simulink model "BCM2_4"  (R2021b)
settings: Solver=FixedStepDiscrete  StartTime=0.0  StopTime=1  FixedStep=0.001  RelTol=1e-3  EnableMultiTasking=on
InitFcn:
  | mbd_mpc_consistency_checks(bdroot(gcs));
model workspace (MAT data in the model file):
  CAN_rec : Simulink.Signal (value not decoded)
  CAN_transm_stat : Simulink.Signal (value not decoded)
  CAN_trm : Simulink.Signal (value not decoded)
  DITHER_CFB0 : Simulink.Parameter (value not decoded)
  DITHER_CFB1 : Simulink.Parameter (value not decoded)
  DITHER_CFB2 : Simulink.Parameter (value not decoded)
  DITHER_EN0 : Simulink.Parameter (value not decoded)
  DITHER_EN1 : Simulink.Parameter (value not decoded)
  DITHER_EN2 : Simulink.Parameter (value not decoded)
  DITHER_SIZE0 : Simulink.Parameter (value not decoded)
  DITHER_SIZE1 : Simulink.Parameter (value not decoded)
  DITHER_SIZE2 : Simulink.Parameter (value not decoded)
  DITHER_STEP0 : Simulink.Parameter (value not decoded)
  DITHER_STEP1 : Simulink.Parameter (value not decoded)
  DITHER_STEP2 : Simulink.Parameter (value not decoded)
  DITHER_SYNC0 : Simulink.Parameter (value not decoded)
  DITHER_SYNC1 : Simulink.Parameter (value not decoded)
  DITHER_SYNC2 : Simulink.Parameter (value not decoded)
  ECUMbut : Simulink.Signal (value not decoded)
  FAULTN : Simulink.Signal (value not decoded)
  FM0 : Simulink.Parameter (value not decoded)
  FM1 : Simulink.Parameter (value not decoded)
  FM2 : Simulink.Parameter (value not decoded)
  FME : Simulink.Parameter (value not decoded)
  Fsys_M : Simulink.Parameter (value not decoded)
  Fsys_N : Simulink.Parameter (value not decoded)
  Fsys_WDEN : Simulink.Parameter (value not decoded)
  Fsys_div : Simulink.Parameter (value not decoded)
  HL0 : Simulink.Parameter (value not decoded)
  HL1 : Simulink.Parameter (value not decoded)
  HL2 : Simulink.Parameter (value not decoded)
  IDIAG0 : Simulink.Parameter (value not decoded)
  IDIAG1 : Simulink.Parameter (value not decoded)
  IDIAG2 : Simulink.Parameter (value not decoded)
  Ivalve : Simulink.Signal (value not decoded)
  KI_index0 : Simulink.Parameter (value not decoded)
  KI_index1 : Simulink.Parameter (value not decoded)
  KI_index2 : Simulink.Parameter (value not decoded)
  PWM_Period0 : Simulink.Parameter (value not decoded)
  PWM_Period1 : Simulink.Parameter (value not decoded)
  PWM_Period2 : Simulink.Parameter (value not decoded)
  RESN : Simulink.Signal (value not decoded)
  SR0 : Simulink.Parameter (value not decoded)
  SR1 : Simulink.Parameter (value not decoded)
  SR2 : Simulink.Parameter (value not decoded)
  Vparam : Simulink.Signal (value not decoded)
  block_tle : Simulink.Signal (value not decoded)
  disp : Simulink.Signal (value not decoded)
  ee_adr : Simulink.Signal (value not decoded)
  ee_en_rd : Simulink.Signal (value not decoded)
  ee_en_wr : Simulink.Signal (value not decoded)
  ee_idle : Simulink.Signal (value not decoded)
  ee_read : Simulink.Signal (value not decoded)
  ee_recv : Simulink.Signal (value not decoded)
  ee_send : Simulink.Signal (value not decoded)
  in_stats : Simulink.Signal (value not decoded)
  inputs : Simulink.Signal (value not decoded)
  light : Simulink.Signal (value not decoded)
  out_drv : Simulink.Signal (value not decoded)
  out_drv_test : Simulink.Signal (value not decoded)
  out_test_en : Simulink.Signal (value not decoded)
  recv_spi2 : Simulink.Signal (value not decoded)
  ret : Simulink.Signal (value not decoded)
  spi_rcv_tle82453 : Simulink.Signal (value not decoded)
  tle82453_Ivlv : Simulink.Signal (value not decoded)
  tle82453_err : Simulink.Signal (value not decoded)
  tle82453_reset : Simulink.Signal (value not decoded)
  wtdg_CAN : Simulink.Signal (value not decoded)
symbols that are objects in the model workspace (value not decoded): CAN_rec, CAN_transm_stat, ECUMbut, inputs, Ivalve, out_drv_test, recv_spi2, ret, SR0, tle82453_Ivlv
undefined symbols (not defined in the file or in its folder): color, LQFP
libraries: simulink x68, mbd_mpc574x_ec_toolbox x50, canmsglib x42, hdlsllib x9, commutil2 x7, etargetslib x4
(part 3 of 6)

== system BCM2_4/Степы ретардера/страницы механика+ ==
  Trigger : TriggerPort  VariantControl=(inherit)
  AND : Logic  AllPortsSameDT=off  OutDataTypeStr=boolean
  AND1 : Logic  AllPortsSameDT=off  OutDataTypeStr=boolean
  Data Store Read : DataStoreRead  DataStoreName=ret  DataStoreElements=ret.step  IndexOptions=Index vector (dialog)  Indices=1  OutputSizes=1
  Data Store Read1 : DataStoreRead  DataStoreName=ret  DataStoreElements=ret.step_brk  IndexOptions=Index vector (dialog)  Indices=1  OutputSizes=1
  Data Store Read2 : DataStoreRead  DataStoreName=ret  DataStoreElements=ret.stat_ret_brk  IndexOptions=Index vector (dialog)  Indices=1  OutputSizes=1
  Max_step : Constant  Value=5  OutDataTypeStr=uint8
  Max_step1 : Constant  Value=3  OutDataTypeStr=uint8
  NOT1 : Logic  Operator=NOT  IconShape=distinctive  AllPortsSameDT=off  OutDataTypeStr=boolean
  Relational Operator : RelationalOperator  Operator=>  OutDataTypeStr=boolean  RndMeth=Simplest
  Relational Operator1 : RelationalOperator  Operator=>  OutDataTypeStr=boolean  RndMeth=Simplest
  Subsystem : Subsystem
  Subsystem1 : Subsystem
  Out_max_ret : Outport
  Out_max_brk : Outport  Port=2
  wires:
  Relational Operator/1 -> AND/1
  Data Store Read/1 -> Relational Operator/2
  Max_step/1 -> Out_max_ret/1, Relational Operator/1
  Max_step1/1 -> Relational Operator1/1, Out_max_brk/1
  Data Store Read1/1 -> Relational Operator1/2
  Relational Operator1/1 -> AND1/1
  AND/1 -> Subsystem/Enable
  AND1/1 -> Subsystem1/Enable
  Data Store Read2/1 -> AND1/2, NOT1/1
  NOT1/1 -> AND/2

== system BCM2_4/Степы ретардера/страницы механика- ==
  Trigger : TriggerPort  VariantControl=(inherit)
  Constant : Constant  Value=2
  Data Store Read1 : DataStoreRead  DataStoreName=ret  DataStoreElements=ret.step  IndexOptions=Index vector (dialog)  Indices=1  OutputSizes=1
  Relational Operator : RelationalOperator  Operator=>  OutDataTypeStr=boolean  RndMeth=Simplest
  Subsystem : Subsystem
  wires:
  Constant/1 -> Relational Operator/2
  Data Store Read1/1 -> Relational Operator/1
  Relational Operator/1 -> Subsystem/Enable

== system BCM2_4/Топливные баки/Enabled Subsystem ==
  Enable : EnablePort
  Compare To Constant : simulink/Logic and Bit Operations/Compare To Constant  relop=>=  const=0.8  OutDataTypeStr=boolean
  Data Store Read : DataStoreRead  DataStoreName=tank1  IndexOptions=Index vector (dialog)  Indices=1  OutputSizes=1
  Subsystem : Subsystem
  wires:
  Data Store Read/1 -> Compare To Constant/1
  Compare To Constant/1 -> Subsystem/Enable

== system BCM2_4/Топливные баки/Enabled Subsystem1 ==
  Enable : EnablePort
  Compare To Constant : simulink/Logic and Bit Operations/Compare To Constant  relop=>=  const=0.8  OutDataTypeStr=boolean
  Data Store Read : DataStoreRead  DataStoreName=tank2  IndexOptions=Index vector (dialog)  Indices=1  OutputSizes=1
  Subsystem : Subsystem
  wires:
  Compare To Constant/1 -> Subsystem/Enable
  Data Store Read/1 -> Compare To Constant/1

== system BCM2_4/Топливные баки/Subsystem ==
  In1 : Inport
  Enable : EnablePort
  Add1 : Sum  Inputs=+-
  Data Store Read1 : DataStoreRead  DataStoreName=tank3  SampleTime=1  IndexOptions=Index vector (dialog)  Indices=1  OutputSizes=1
  Data Store Write1 : DataStoreWrite  DataStoreName=tank3  IndexOptions=Index vector (dialog)  Indices=1  OutputSizes=1
  wires:
  Data Store Read1/1 -> Add1/1
  Add1/1 -> Data Store Write1/1
  In1/1 -> Add1/2

== system BCM2_4/Управление с клавиатуры ECUMASTER/1 ==
  PM_up : Inport
  Trigger : TriggerPort  TriggerType=either  VariantControl=(inherit)  PortDimensions=1
  Data Store Write3 : DataStoreWrite  DataStoreName=ECUMbut  DataStoreElements=ECUMbut.win_Up_Pilot  IndexOptions=Index vector (dialog)  Indices=1  OutputSizes=1
  Data Type Conversion : DataTypeConversion  OutDataTypeStr=uint8
  Enumerated Constant : simulink/Sources/Enumerated Constant  OutDataTypeStr=Enum: color  Value=color.orange  SampleTime=inf
  Enumerated Constant1 : simulink/Sources/Enumerated Constant  OutDataTypeStr=Enum: color  Value=color.off  SampleTime=inf
  Switch : Switch  Criteria=u2 > Threshold
  Out1 : Outport
  wires:
  Data Type Conversion/1 -> Out1/1
  Enumerated Constant1/1 -> Switch/3
  Enumerated Constant/1 -> Switch/1
  Switch/1 -> Data Type Conversion/1
  PM_up/1 -> Switch/2, Data Store Write3/1

== system BCM2_4/Управление с клавиатуры ECUMASTER/2 ==
  PM_up : Inport
  Trigger : TriggerPort  TriggerType=either  VariantControl=(inherit)  PortDimensions=1
  Data Store Write3 : DataStoreWrite  DataStoreName=ECUMbut  DataStoreElements=ECUMbut.win_Dn_Pilot  IndexOptions=Index vector (dialog)  Indices=1  OutputSizes=1
  Data Type Conversion : DataTypeConversion  OutDataTypeStr=uint8
  Enumerated Constant : simulink/Sources/Enumerated Constant  OutDataTypeStr=Enum: color  Value=color.orange  SampleTime=inf
  Enumerated Constant1 : simulink/Sources/Enumerated Constant  OutDataTypeStr=Enum: color  Value=color.off  SampleTime=inf
  Switch : Switch  Criteria=u2 > Threshold
  Out1 : Outport
  wires:
  PM_up/1 -> Data Store Write3/1, Switch/2
  Switch/1 -> Data Type Conversion/1
  Enumerated Constant/1 -> Switch/1
  Enumerated Constant1/1 -> Switch/3
  Data Type Conversion/1 -> Out1/1

== system BCM2_4/Управление с клавиатуры ECUMASTER/3 ==
  PM_up : Inport
  Trigger : TriggerPort  TriggerType=either  VariantControl=(inherit)  PortDimensions=1
  Data Store Write3 : DataStoreWrite  DataStoreName=ECUMbut  DataStoreElements=ECUMbut.win_Up_Meh  IndexOptions=Index vector (dialog)  Indices=1  OutputSizes=1
  Data Type Conversion : DataTypeConversion  OutDataTypeStr=uint8
  Enumerated Constant : simulink/Sources/Enumerated Constant  OutDataTypeStr=Enum: color  Value=color.orange  SampleTime=inf
  Enumerated Constant1 : simulink/Sources/Enumerated Constant  OutDataTypeStr=Enum: color  Value=color.off  SampleTime=inf
  Switch : Switch  Criteria=u2 > Threshold
  Out1 : Outport
  wires:
  Data Type Conversion/1 -> Out1/1
  Enumerated Constant1/1 -> Switch/3
  Enumerated Constant/1 -> Switch/1
  Switch/1 -> Data Type Conversion/1
  PM_up/1 -> Switch/2, Data Store Write3/1

== system BCM2_4/Управление с клавиатуры ECUMASTER/4 ==
  PM_up : Inport
  Trigger : TriggerPort  TriggerType=either  VariantControl=(inherit)  PortDimensions=1
  Data Store Write3 : DataStoreWrite  DataStoreName=ECUMbut  DataStoreElements=ECUMbut.win_Dn_Meh  IndexOptions=Index vector (dialog)  Indices=1  OutputSizes=1
  Data Type Conversion : DataTypeConversion  OutDataTypeStr=uint8
  Enumerated Constant : simulink/Sources/Enumerated Constant  OutDataTypeStr=Enum: color  Value=color.orange  SampleTime=inf
  Enumerated Constant1 : simulink/Sources/Enumerated Constant  OutDataTypeStr=Enum: color  Value=color.off  SampleTime=inf
  Switch : Switch  Criteria=u2 > Threshold
  Out1 : Outport
  wires:
  PM_up/1 -> Data Store Write3/1, Switch/2
  Switch/1 -> Data Type Conversion/1
  Enumerated Constant/1 -> Switch/1
  Enumerated Constant1/1 -> Switch/3
  Data Type Conversion/1 -> Out1/1

== system BCM2_4/Управление с клавиатуры ECUMASTER/Check АКП ==
  In1 : Inport
  Trigger : TriggerPort  TriggerType=either  VariantControl=(inherit)  PortDimensions=1
  Data Store Write3 : DataStoreWrite  DataStoreName=ECUMbut  DataStoreElements=ECUMbut.check_AT  IndexOptions=Index vector (dialog)  Indices=1  OutputSizes=1
  Data Type Conversion : DataTypeConversion  OutDataTypeStr=uint8
  Enumerated Constant : simulink/Sources/Enumerated Constant  OutDataTypeStr=Enum: color  Value=color.orange  SampleTime=inf
  Enumerated Constant1 : simulink/Sources/Enumerated Constant  OutDataTypeStr=Enum: color  Value=color.off  SampleTime=inf
  Switch : Switch  Criteria=u2 > Threshold
  Out1 : Outport
  wires:
  In1/1 -> Data Store Write3/1, Switch/2
  Switch/1 -> Data Type Conversion/1
  Enumerated Constant/1 -> Switch/1
  Enumerated Constant1/1 -> Switch/3
  Data Type Conversion/1 -> Out1/1

== system BCM2_4/Управление с клавиатуры ECUMASTER/Enabled Subsystem ==
  left : Inport
  right : Inport  Port=2
  hazard : Inport  Port=3
  Enable : EnablePort
  AND : Logic  AllPortsSameDT=off  OutDataTypeStr=boolean
  AND1 : Logic  AllPortsSameDT=off  OutDataTypeStr=boolean
  AND2 : Logic  AllPortsSameDT=off  OutDataTypeStr=boolean
  Data Type Conversion : DataTypeConversion  OutDataTypeStr=uint8
  Discrete Pulse Generator : DiscretePulseGenerator  Period=60  PulseWidth=20  SampleTime=-1
  Enumerated Constant : simulink/Sources/Enumerated Constant  OutDataTypeStr=Enum: color  Value=color.red  SampleTime=inf
  Enumerated Constant1 : simulink/Sources/Enumerated Constant  OutDataTypeStr=Enum: color  Value=color.off  SampleTime=inf
  OR : Logic  Operator=OR  AllPortsSameDT=off  OutDataTypeStr=boolean
  OR1 : Logic  Operator=OR  AllPortsSameDT=off  OutDataTypeStr=boolean
  Switch : Switch  Criteria=u2 > Threshold
  Out1 : Outport  OutputWhenDisabled=reset  InitialOutput=0
  Out2 : Outport  Port=2  OutputWhenDisabled=reset  InitialOutput=0
  Out3 : Outport  Port=3  OutputWhenDisabled=reset  InitialOutput=0
  wires:
  left/1 -> OR/1
  AND/1 -> Out2/1
  Discrete Pulse Generator/1 -> AND2/1, AND1/1, AND/2
  AND1/1 -> Out3/1
  OR/1 -> AND/1
  OR1/1 -> AND1/2
  Enumerated Constant1/1 -> Switch/3
  Enumerated Constant/1 -> Switch/1
  AND2/1 -> Switch/2
  Switch/1 -> Data Type Conversion/1
  Data Type Conversion/1 -> Out1/1
  right/1 -> OR1/2
  hazard/1 -> AND2/2, OR/2, OR1/1

== system BCM2_4/Управление с клавиатуры ECUMASTER/Вентилятор пилота ==
  Trigger : TriggerPort  VariantControl=(inherit)  PortDimensions=1
  Data Store Read1 : DataStoreRead  DataStoreName=ECUMbut  DataStoreElements=ECUMbut.fan  IndexOptions=Index vector (dialog)  Indices=1  OutputSizes=1
  Data Store Read4 : DataStoreRead  DataStoreName=ECUMbut  DataStoreElements=ECUMbut.fan  IndexOptions=Index vector (dialog)  Indices=1  OutputSizes=1
  Data Store Write3 : DataStoreWrite  DataStoreName=ECUMbut  DataStoreElements=ECUMbut.fan  IndexOptions=Index vector (dialog)  Indices=1  OutputSizes=1
  Data Type Conversion : DataTypeConversion  OutDataTypeStr=uint8
  Enumerated Constant : simulink/Sources/Enumerated Constant  OutDataTypeStr=Enum: color  Value=color.red  SampleTime=inf
  Enumerated Constant1 : simulink/Sources/Enumerated Constant  OutDataTypeStr=Enum: color  Value=color.off  SampleTime=inf
  NOT : Logic  Operator=NOT  IconShape=distinctive  AllPortsSameDT=off  OutDataTypeStr=boolean
  Switch : Switch  Criteria=u2 > Threshold
  Out1 : Outport
  wires:
  NOT/1 -> Data Store Write3/1
  Data Store Read4/1 -> NOT/1
  Switch/1 -> Data Type Conversion/1
  Enumerated Constant/1 -> Switch/1
  Enumerated Constant1/1 -> Switch/3
  Data Type Conversion/1 -> Out1/1
  Data Store Read1/1 -> Switch/2

== system BCM2_4/Управление с клавиатуры ECUMASTER/Обогрев лобового стекла ==
  Trigger : TriggerPort  VariantControl=(inherit)  PortDimensions=1
  Data Store Read1 : DataStoreRead  DataStoreName=ECUMbut  DataStoreElements=ECUMbut.heat  IndexOptions=Index vector (dialog)  Indices=1  OutputSizes=1
  Data Store Read4 : DataStoreRead  DataStoreName=ECUMbut  DataStoreElements=ECUMbut.heat  IndexOptions=Index vector (dialog)  Indices=1  OutputSizes=1
  Data Store Write3 : DataStoreWrite  DataStoreName=ECUMbut  DataStoreElements=ECUMbut.heat  IndexOptions=Index vector (dialog)  Indices=1  OutputSizes=1
  Data Type Conversion : DataTypeConversion  OutDataTypeStr=uint8
  Enumerated Constant : simulink/Sources/Enumerated Constant  OutDataTypeStr=Enum: color  Value=color.green  SampleTime=inf
  Enumerated Constant1 : simulink/Sources/Enumerated Constant  OutDataTypeStr=Enum: color  Value=color.off  SampleTime=inf
  NOT : Logic  Operator=NOT  IconShape=distinctive  AllPortsSameDT=off  OutDataTypeStr=boolean
  Switch : Switch  Criteria=u2 > Threshold
  Out1 : Outport
  wires:
  Data Type Conversion/1 -> Out1/1
  Enumerated Constant1/1 -> Switch/3
  Enumerated Constant/1 -> Switch/1
  Switch/1 -> Data Type Conversion/1
  Data Store Read4/1 -> NOT/1
  NOT/1 -> Data Store Write3/1
  Data Store Read1/1 -> Switch/2

== system BCM2_4/Управление с клавиатуры ECUMASTER/Переключение таблиц ДВС ==
  Trigger : TriggerPort  VariantControl=(inherit)
  Add : Sum
  Compare To Constant : simulink/Logic and Bit Operations/Compare To Constant  Priority=6  relop=>  const=2  OutDataTypeStr=boolean
  Constant : Constant  OutDataTypeStr=uint8
  Data Store Read1 : DataStoreRead  Priority=1  DataStoreName=ECUMbut  DataStoreElements=ECUMbut.cnt(2)  IndexOptions=Index vector (dialog)  Indices=1  OutputSizes=1
  Data Store Read2 : DataStoreRead  Priority=4  DataStoreName=ECUMbut  DataStoreElements=ECUMbut.cnt(2)  IndexOptions=Index vector (dialog)  Indices=1  OutputSizes=1
  Data Store Read3 : DataStoreRead  Priority=8  DataStoreName=ECUMbut  DataStoreElements=ECUMbut.cnt(2)  IndexOptions=Index vector (dialog)  Indices=1  OutputSizes=1
  Data Store Write1 : DataStoreWrite  DataStoreName=ECUMbut  DataStoreElements=ECUMbut.cnt(2)  IndexOptions=Index vector (dialog)  Indices=1  OutputSizes=1
  Data Store Write2 : DataStoreWrite  DataStoreName=ECUMbut  DataStoreElements=ECUMbut.table_rom  IndexOptions=Index vector (dialog)  Indices=1  OutputSizes=1
  Data Type Conversion : DataTypeConversion  OutDataTypeStr=uint8
  Enumerated Constant : simulink/Sources/Enumerated Constant  OutDataTypeStr=Enum: color  Value=color.off  SampleTime=inf
  Enumerated Constant2 : simulink/Sources/Enumerated Constant  OutDataTypeStr=Enum: color  Value=color.red  SampleTime=inf
  Enumerated Constant3 : simulink/Sources/Enumerated Constant  OutDataTypeStr=Enum: color  Value=color.blue  SampleTime=inf
  Multiport Switch : MultiPortSwitch  DataPortOrder=Zero-based contiguous  zeroidx=on
  сброс на ноль : Subsystem
  Out1 : Outport
  wires:
  Multiport Switch/1 -> Data Type Conversion/1
  Enumerated Constant3/1 -> Multiport Switch/4
  Enumerated Constant2/1 -> Multiport Switch/3
  Enumerated Constant/1 -> Multiport Switch/2
  Data Type Conversion/1 -> Out1/1
  Add/1 -> Data Store Write1/1
  Constant/1 -> Add/2
  Data Store Read1/1 -> Add/1
  Compare To Constant/1 -> сброс на ноль/Enable
  Data Store Read2/1 -> Data Store Write2/1, Compare To Constant/1
  Data Store Read3/1 -> Multiport Switch/1

== system BCM2_4/Управление с клавиатуры ECUMASTER/Страницы пилота+ ==
  In1 : Inport
  Trigger : TriggerPort  TriggerType=either  VariantControl=(inherit)  PortDimensions=1
  Data Store Write3 : DataStoreWrite  DataStoreName=ECUMbut  DataStoreElements=ECUMbut.PageP  IndexOptions=Index vector (dialog)  Indices=1  OutputSizes=1
  Data Type Conversion : DataTypeConversion  OutDataTypeStr=uint8
  Enumerated Constant : simulink/Sources/Enumerated Constant  OutDataTypeStr=Enum: color  Value=color.white  SampleTime=inf
  Enumerated Constant1 : simulink/Sources/Enumerated Constant  OutDataTypeStr=Enum: color  Value=color.off  SampleTime=inf
  Switch : Switch  Criteria=u2 > Threshold
  Out1 : Outport
  wires:
  In1/1 -> Data Store Write3/1, Switch/2
  Switch/1 -> Data Type Conversion/1
  Enumerated Constant/1 -> Switch/1
  Enumerated Constant1/1 -> Switch/3
  Data Type Conversion/1 -> Out1/1

== system BCM2_4/Управление с клавиатуры ECUMASTER/Страницы пилота- ==
  In1 : Inport
  Trigger : TriggerPort  TriggerType=either  VariantControl=(inherit)  PortDimensions=1
  Data Store Write3 : DataStoreWrite  DataStoreName=ECUMbut  DataStoreElements=ECUMbut.PageM  IndexOptions=Index vector (dialog)  Indices=1  OutputSizes=1
  Data Type Conversion : DataTypeConversion  OutDataTypeStr=uint8
  Enumerated Constant : simulink/Sources/Enumerated Constant  OutDataTypeStr=Enum: color  Value=color.white  SampleTime=inf
  Enumerated Constant1 : simulink/Sources/Enumerated Constant  OutDataTypeStr=Enum: color  Value=color.off  SampleTime=inf
  Switch : Switch  Criteria=u2 > Threshold
  Out1 : Outport
  wires:
  Data Type Conversion/1 -> Out1/1
  Enumerated Constant1/1 -> Switch/3
  Enumerated Constant/1 -> Switch/1
  Switch/1 -> Data Type Conversion/1
  In1/1 -> Switch/2, Data Store Write3/1

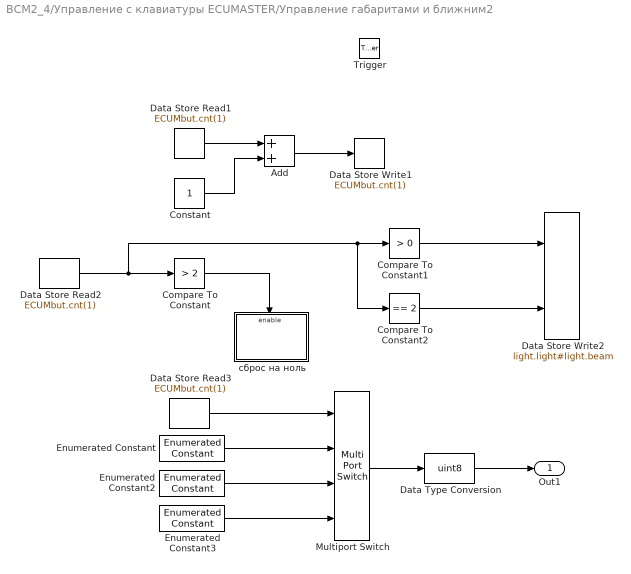
== system BCM2_4/Управление с клавиатуры ECUMASTER/Управление габаритами и ближним2 ==
  Trigger : TriggerPort  VariantControl=(inherit)
  Add : Sum
  Compare To Constant : simulink/Logic and Bit Operations/Compare To Constant  relop=>  const=2  OutDataTypeStr=boolean
  Compare To Constant1 : simulink/Logic and Bit Operations/Compare To Constant  relop=>  const=0  OutDataTypeStr=boolean
  Compare To Constant2 : simulink/Logic and Bit Operations/Compare To Constant  relop===  const=2  OutDataTypeStr=boolean
  Constant : Constant  OutDataTypeStr=uint8
  Data Store Read1 : DataStoreRead  Priority=1  DataStoreName=ECUMbut  DataStoreElements=ECUMbut.cnt(1)  IndexOptions=Index vector (dialog)  Indices=1  OutputSizes=1
  Data Store Read2 : DataStoreRead  Priority=7  DataStoreName=ECUMbut  DataStoreElements=ECUMbut.cnt(1)  IndexOptions=Index vector (dialog)  Indices=1  OutputSizes=1
  Data Store Read3 : DataStoreRead  Priority=8  DataStoreName=ECUMbut  DataStoreElements=ECUMbut.cnt(1)  IndexOptions=Index vector (dialog)  Indices=1  OutputSizes=1
  Data Store Write1 : DataStoreWrite  DataStoreName=ECUMbut  DataStoreElements=ECUMbut.cnt(1)  IndexOptions=Index vector (dialog)  Indices=1  OutputSizes=1
  Data Store Write2 : DataStoreWrite  DataStoreName=light  DataStoreElements=light.light#light.beam  IndexOptions=Index vector (dialog)  Indices=1  OutputSizes=1
  Data Type Conversion : DataTypeConversion  OutDataTypeStr=uint8
  Enumerated Constant : simulink/Sources/Enumerated Constant  OutDataTypeStr=Enum: color  Value=color.off  SampleTime=inf
  Enumerated Constant2 : simulink/Sources/Enumerated Constant  OutDataTypeStr=Enum: color  Value=color.green  SampleTime=inf
  Enumerated Constant3 : simulink/Sources/Enumerated Constant  OutDataTypeStr=Enum: color  Value=color.blue  SampleTime=inf
  Multiport Switch : MultiPortSwitch  DataPortOrder=Zero-based contiguous  zeroidx=on
  сброс на ноль : Subsystem
  Out1 : Outport
  wires:
  Data Type Conversion/1 -> Out1/1
  Data Store Read3/1 -> Multiport Switch/1
  Data Store Read2/1 -> Compare To Constant2/1, Compare To Constant1/1, Compare To Constant/1
  Compare To Constant/1 -> сброс на ноль/Enable
  Data Store Read1/1 -> Add/1
  Constant/1 -> Add/2
  Add/1 -> Data Store Write1/1
  Compare To Constant1/1 -> Data Store Write2/1
  Compare To Constant2/1 -> Data Store Write2/2
  Multiport Switch/1 -> Data Type Conversion/1
  Enumerated Constant/1 -> Multiport Switch/2
  Enumerated Constant2/1 -> Multiport Switch/3
  Enumerated Constant3/1 -> Multiport Switch/4

== system BCM2_4/Управление с клавиатуры ECUMASTER/Электросигнал ==
  In1 : Inport
  Trigger : TriggerPort  TriggerType=either  VariantControl=(inherit)  PortDimensions=1
  Data Store Write3 : DataStoreWrite  DataStoreName=ECUMbut  DataStoreElements=ECUMbut.horn  IndexOptions=Index vector (dialog)  Indices=1  OutputSizes=1
  Data Type Conversion : DataTypeConversion  OutDataTypeStr=uint8
  Enumerated Constant : simulink/Sources/Enumerated Constant  OutDataTypeStr=Enum: color  Value=color.orange  SampleTime=inf
  Enumerated Constant1 : simulink/Sources/Enumerated Constant  OutDataTypeStr=Enum: color  Value=color.off  SampleTime=inf
  Switch : Switch  Criteria=u2 > Threshold
  Out1 : Outport
  wires:
  Data Type Conversion/1 -> Out1/1
  Enumerated Constant1/1 -> Switch/3
  Enumerated Constant/1 -> Switch/1
  Switch/1 -> Data Type Conversion/1
  In1/1 -> Switch/2, Data Store Write3/1

== system BCM2_4/Управление с клавиатуры ECUMASTER/Яркость пилота ==
  Trigger : TriggerPort  VariantControl=(inherit)  PortDimensions=1
  Data Store Read1 : DataStoreRead  DataStoreName=ECUMbut  DataStoreElements=ECUMbut.bright_pilot  IndexOptions=Index vector (dialog)  Indices=1  OutputSizes=1
  Data Store Read4 : DataStoreRead  DataStoreName=ECUMbut  DataStoreElements=ECUMbut.bright_pilot  IndexOptions=Index vector (dialog)  Indices=1  OutputSizes=1
  Data Store Write3 : DataStoreWrite  DataStoreName=ECUMbut  DataStoreElements=ECUMbut.bright_pilot  IndexOptions=Index vector (dialog)  Indices=1  OutputSizes=1
  Data Type Conversion : DataTypeConversion  OutDataTypeStr=uint8
  Enumerated Constant : simulink/Sources/Enumerated Constant  OutDataTypeStr=Enum: color  Value=color.bluegreen  SampleTime=inf
  Enumerated Constant1 : simulink/Sources/Enumerated Constant  OutDataTypeStr=Enum: color  Value=color.off  SampleTime=inf
  NOT : Logic  Operator=NOT  IconShape=distinctive  AllPortsSameDT=off  OutDataTypeStr=boolean
  Switch : Switch  Criteria=u2 > Threshold
  Out1 : Outport
  wires:
  Data Type Conversion/1 -> Out1/1
  Enumerated Constant1/1 -> Switch/3
  Enumerated Constant/1 -> Switch/1
  Switch/1 -> Data Type Conversion/1
  Data Store Read4/1 -> NOT/1
  NOT/1 -> Data Store Write3/1
  Data Store Read1/1 -> Switch/2

== system BCM2_4/Управление с клавиатуры ECUMASTER/включение аварийки ==
  Trigger : TriggerPort  VariantControl=(inherit)  PortDimensions=1
  Data Store Read4 : DataStoreRead  DataStoreName=ECUMbut  DataStoreElements=ECUMbut.hazard  IndexOptions=Index vector (dialog)  Indices=1  OutputSizes=1
  Data Store Write3 : DataStoreWrite  DataStoreName=ECUMbut  DataStoreElements=ECUMbut.hazard  IndexOptions=Index vector (dialog)  Indices=1  OutputSizes=1
  NOT : Logic  Operator=NOT  IconShape=distinctive  AllPortsSameDT=off  OutDataTypeStr=boolean
  wires:
  Data Store Read4/1 -> NOT/1
  NOT/1 -> Data Store Write3/1

== system BCM2_4/Управление с клавиатуры ECUMASTER/включение допов ==
  Trigger : TriggerPort  VariantControl=(inherit)  PortDimensions=1
  Data Store Read1 : DataStoreRead  DataStoreName=light  DataStoreElements=light.dop  IndexOptions=Index vector (dialog)  Indices=1  OutputSizes=1
  Data Store Read4 : DataStoreRead  DataStoreName=light  DataStoreElements=light.dop  IndexOptions=Index vector (dialog)  Indices=1  OutputSizes=1
  Data Store Write3 : DataStoreWrite  DataStoreName=light  DataStoreElements=light.dop  IndexOptions=Index vector (dialog)  Indices=1  OutputSizes=1
  Data Type Conversion : DataTypeConversion  OutDataTypeStr=uint8
  Enumerated Constant : simulink/Sources/Enumerated Constant  OutDataTypeStr=Enum: color  Value=color.blue  SampleTime=inf
  Enumerated Constant1 : simulink/Sources/Enumerated Constant  OutDataTypeStr=Enum: color  Value=color.off  SampleTime=inf
  NOT : Logic  Operator=NOT  IconShape=distinctive  AllPortsSameDT=off  OutDataTypeStr=boolean
  Switch : Switch  Criteria=u2 > Threshold
  Out1 : Outport
  wires:
  NOT/1 -> Data Store Write3/1
  Data Store Read4/1 -> NOT/1
  Switch/1 -> Data Type Conversion/1
  Enumerated Constant/1 -> Switch/1
  Enumerated Constant1/1 -> Switch/3
  Data Type Conversion/1 -> Out1/1
  Data Store Read1/1 -> Switch/2

== system BCM2_4/Управление с клавиатуры ECUMASTER/включение подпирающего топливного насоса ==
  Trigger : TriggerPort  VariantControl=(inherit)  PortDimensions=1
  Data Store Read1 : DataStoreRead  DataStoreName=ECUMbut  DataStoreElements=ECUMbut.pump  IndexOptions=Index vector (dialog)  Indices=1  OutputSizes=1
  Data Store Read4 : DataStoreRead  DataStoreName=ECUMbut  DataStoreElements=ECUMbut.pump  IndexOptions=Index vector (dialog)  Indices=1  OutputSizes=1
  Data Store Write3 : DataStoreWrite  DataStoreName=ECUMbut  DataStoreElements=ECUMbut.pump  IndexOptions=Index vector (dialog)  Indices=1  OutputSizes=1
  Data Type Conversion : DataTypeConversion  OutDataTypeStr=uint8
  Enumerated Constant : simulink/Sources/Enumerated Constant  OutDataTypeStr=Enum: color  Value=color.bluegreen  SampleTime=inf
  Enumerated Constant1 : simulink/Sources/Enumerated Constant  OutDataTypeStr=Enum: color  Value=color.off  SampleTime=inf
  NOT : Logic  Operator=NOT  IconShape=distinctive  AllPortsSameDT=off  OutDataTypeStr=boolean
  Switch : Switch  Criteria=u2 > Threshold
  Out1 : Outport
  wires:
  NOT/1 -> Data Store Write3/1
  Data Store Read4/1 -> NOT/1
  Switch/1 -> Data Type Conversion/1
  Enumerated Constant/1 -> Switch/1
  Enumerated Constant1/1 -> Switch/3
  Data Type Conversion/1 -> Out1/1
  Data Store Read1/1 -> Switch/2

== system BCM2_4/назначение входов и выходов/диагностика выходов ==
  Enable : EnablePort
  Data Store Read4 : DataStoreRead  DataStoreName=CAN_rec  DataStoreElements=CAN_rec.ee_data  IndexOptions=Index vector (dialog)  Indices=1  OutputSizes=1
  Data Store Write3 : DataStoreWrite  DataStoreName=out_drv_test  IndexOptions=Index vector (dialog)  Indices=1  OutputSizes=1
  Integer to Bit Converter1 : commutil2/Integer to Bit Converter  nbits=16  signedInputValues=Unsigned  bitOrder=LSB first  outDtype=boolean
  wires:
  Integer to Bit Converter1/1 -> Data Store Write3/1
  Data Store Read4/1 -> Integer to Bit Converter1/1

== system BCM2_4/управление страницами и яркостью мониторов/страницы механика+ ==
  Trigger : TriggerPort  VariantControl=(inherit)
  Data Store Read : DataStoreRead  DataStoreName=disp  DataStoreElements=disp.meh_max_page#disp.meh_page  IndexOptions=Index vector (dialog)  Indices=1  OutputSizes=1
  Relational Operator : RelationalOperator  Operator=>  OutDataTypeStr=boolean  RndMeth=Simplest
  Subsystem : Subsystem
  wires:
  Relational Operator/1 -> Subsystem/Enable
  Data Store Read/2 -> Relational Operator/2
  Data Store Read/1 -> Relational Operator/1

== system BCM2_4/управление страницами и яркостью мониторов/страницы механика- ==
  Trigger : TriggerPort  VariantControl=(inherit)
  Constant : Constant
  Data Store Read1 : DataStoreRead  DataStoreName=disp  DataStoreElements=disp.meh_page  IndexOptions=Index vector (dialog)  Indices=1  OutputSizes=1
  Relational Operator : RelationalOperator  Operator=>  OutDataTypeStr=boolean  RndMeth=Simplest
  Subsystem : Subsystem
  wires:
  Constant/1 -> Relational Operator/2
  Data Store Read1/1 -> Relational Operator/1
  Relational Operator/1 -> Subsystem/Enable

== system BCM2_4/управление страницами и яркостью мониторов/страницы пилота+ ==
  Trigger : TriggerPort  VariantControl=(inherit)
  Data Store Read : DataStoreRead  DataStoreName=disp  DataStoreElements=disp.pilot_max_page#disp.pilot_page  IndexOptions=Index vector (dialog)  Indices=1  OutputSizes=1
  Relational Operator : RelationalOperator  Operator=>  OutDataTypeStr=boolean  RndMeth=Simplest
  Subsystem : Subsystem
  wires:
  Data Store Read/1 -> Relational Operator/1
  Data Store Read/2 -> Relational Operator/2
  Relational Operator/1 -> Subsystem/Enable

== system BCM2_4/управление страницами и яркостью мониторов/страницы пилота- ==
  Trigger : TriggerPort  VariantControl=(inherit)
  Constant : Constant
  Data Store Read1 : DataStoreRead  DataStoreName=disp  DataStoreElements=disp.pilot_page  IndexOptions=Index vector (dialog)  Indices=1  OutputSizes=1
  Relational Operator : RelationalOperator  Operator=>  OutDataTypeStr=boolean  RndMeth=Simplest
  Subsystem : Subsystem
  wires:
  Relational Operator/1 -> Subsystem/Enable
  Data Store Read1/1 -> Relational Operator/1
  Constant/1 -> Relational Operator/2

== system BCM2_4/CAN0 Transmit buf 5-21/0CFED911 AUXIO buf = 11/0CFED911 AUXIO buf = 11 ==
  CAN Pack : canmsglib/CAN Pack  CANdbFile=C:\Temp\j1939.dbc  MsgList=AUXIO  MsgName=AUXIO  MsgIDType=Extended (29-bit identifier)  MsgIdentifier=hex2dec('0CFED911')  MsgLength=8  Remote=off  ApplyMinMax=off  BusOutput=off  SignalInfo={ 'AuxI_O01', '6', '2', 'LE', 'unsigned', 'Standard', '0', '1', '0', '0', '3'; 'AuxI_O02', '4', '2', 'LE', 'unsigned', 'Standard', '0', '1', '0', '0', '3'; 'AuxI_O03', '2', '2', 'LE', 'unsigned', 'Standard', '0', '1', '0', '0', '3'; 'AuxI_O04', '0', '2', 'LE', 'unsigned', 'Standard', '0', '1', '0', '0', '3'; 'AuxI_O05', '14', '2', 'LE', 'unsigned', 'Standard', '0', '1', '0', '0', '3'; 'AuxI_O06', '12', '2', 'LE', 'unsigned', 'Standard', '0', '1', '0', '0', '3'; 'AuxI_O07', '10', '2', 'LE', 'unsigned', 'Standard', '0', '1', '0', '0', '3'; 'AuxI_O08', '8', '2', 'LE', 'unsigned', 'Standard', '0', '1', '0', '0', '3'; 'AuxI_O09', '22', '2', 'LE', 'unsigned', 'Standard', '0', '1', '0', '0', '3'; 'AuxI_O10', '20', '2', 'LE', 'unsigned', 'Standard', '0', '1', '0', '0', '3'; 'AuxI_O11', '18', '2', 'LE', 'unsigned', 'Standard', '0', '1', '0', '0', '3'; 'AuxI_O12', '16', '2', 'LE', 'unsigned', 'Standard', '0', '1', '0', '0', '3'; 'AuxI_O13', '30', '2', 'LE', 'unsigned', 'Standard', '0', '1', '0', '0', '3'; 'AuxI_O14', '28', '2', 'LE', 'unsigned', 'Standard', '0', '1', '0', '0', '3'; 'AuxI_O15', '26', '2', 'LE', 'unsigned', 'Standard', '0', '1', '0', '0', '3'; 'AuxI_O16', '24', '2', 'LE', 'unsigned', 'Standard', '0', '1', '0', '0', '3'; 'AuxI_OChannel1', '32', '16', 'LE', 'unsigned', 'Standard', '0', '1', '0', '0', '64255'; 'AuxI_OChannel2', '48', '16', 'LE', 'unsigned', 'Standard', '0', '1', '0', '0', '64255' }
      settings: SourceProductBaseCode=ME,XP,VN  DataFormat=manually specified signals
  CAN Unpack : canmsglib/CAN Unpack  MsgList=(none)  MsgName=CAN Msg  MsgIDType=Extended (29-bit identifier)  MsgIdentifier=hex2dec('0CFED911')  MsgLength=8  SignalInfo={}  IDPort=off  TimestampPort=off  ErrorPort=off  RemotePort=off  LengthPort=off  StatusPort=off  ApplyMinMax=off
      settings: SourceProductBaseCode=ME,XP,VN  DataFormat=raw data
  Compare To Constant : simulink/Logic and Bit Operations/Compare To Constant  relop===  const=1  OutDataTypeStr=boolean
  Constant4 : Constant  OutDataTypeStr=boolean
  Data Store Read1 : DataStoreRead  DataStoreName=ECUMbut  DataStoreElements=ECUMbut.table_rom  IndexOptions=Index vector (dialog)  Indices=1  OutputSizes=1
  Data Store Read5 : DataStoreRead  DataStoreName=ECUMbut  DataStoreElements=ECUMbut.check_AT  IndexOptions=Index vector (dialog)  Indices=1  OutputSizes=1
  Data Store Write : DataStoreWrite  DataStoreName=CAN_transm_stat  DataStoreElements=CAN_transm_stat(11)  IndexOptions=Index vector (dialog)  Indices=1  OutputSizes=1
  FCAN_Send : mbd_mpc574x_ec_toolbox/Communication Blocks/CAN Blocks/FCAN_Send  Priority=2  can_instance=0  can_mode=Non-blocking  can_timeout_ms=0  can_mb_idx=11  can_extended_id=on  can_is_remote=off  can_id=0CFED911  show_adv_opts=on  can_fd_enable=off  can_enable_brs=off  can_fd_padding=0
      settings: SourceProductName=NXP Model-Based Design Toolbox for MPC57xx MCUs
  Ground : Ground
  Width : Width  DataType=uint8
  wires:
  CAN Pack/1 -> CAN Unpack/1
  CAN Unpack/1 -> FCAN_Send/1, Width/1
  Constant4/1 -> Data Store Write/1
  Width/1 -> FCAN_Send/2
  Data Store Read5/1 -> CAN Pack/5
  Data Store Read1/1 -> Compare To Constant/1
  Compare To Constant/1 -> CAN Pack/1
  Ground/1 -> CAN Pack/17, CAN Pack/16, CAN Pack/15, CAN Pack/14, CAN Pack/13, CAN Pack/12, CAN Pack/11, CAN Pack/10, CAN Pack/9, CAN Pack/8, CAN Pack/7, CAN Pack/6, CAN Pack/2, CAN Pack/3, CAN Pack/4, CAN Pack/18

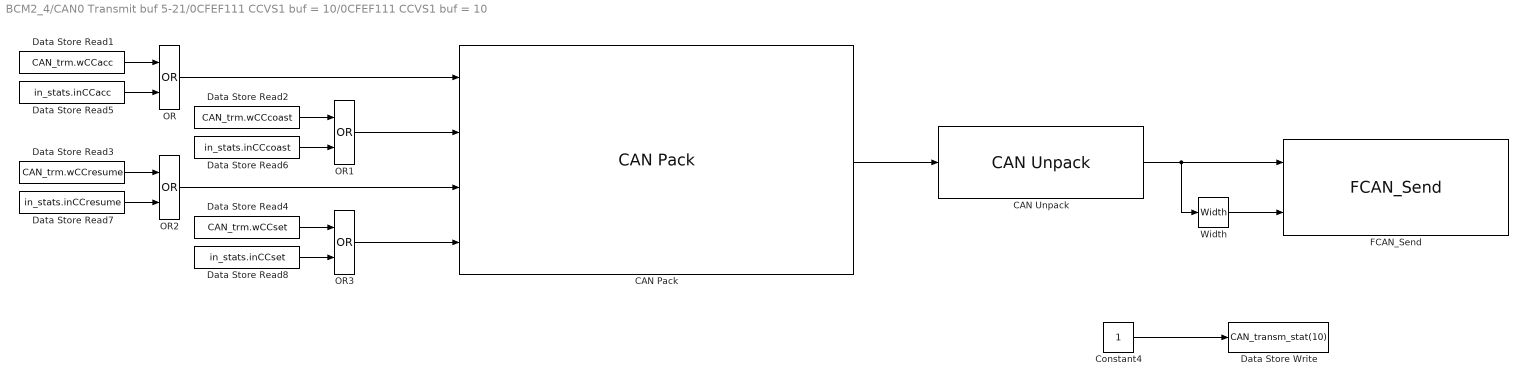
== system BCM2_4/CAN0 Transmit buf 5-21/0CFEF111 CCVS1 buf = 10/0CFEF111 CCVS1 buf = 10 ==
  CAN Pack : canmsglib/CAN Pack  CANdbFile=C:\Temp\j1939.dbc  MsgList=CCVS  MsgName=CCVS  MsgIDType=Extended (29-bit identifier)  MsgIdentifier=hex2dec('0CFEF111')  MsgLength=8  Remote=off  ApplyMinMax=off  BusOutput=off  SignalInfo={ 'CruiseCtrlAccelerateSwitch', '38', '2', 'LE', 'unsigned', 'Standard', '0', '1', '0', '0', '3'; 'CruiseCtrlCoastSwitch', '34', '2', 'LE', 'unsigned', 'Standard', '0', '1', '0', '0', '3'; 'CruiseCtrlResumeSwitch', '36', '2', 'LE', 'unsigned', 'Standard', '0', '1', '0', '0', '3'; 'CruiseCtrlSetSwitch', '32', '2', 'LE', 'unsigned', 'Standard', '0', '1', '0', '0', '3' }
      settings: SourceProductBaseCode=ME,XP,VN  DataFormat=manually specified signals
  CAN Unpack : canmsglib/CAN Unpack  MsgList=(none)  MsgName=CAN Msg  MsgIDType=Extended (29-bit identifier)  MsgIdentifier=hex2dec('0CFEF111')  MsgLength=8  SignalInfo={}  IDPort=off  TimestampPort=off  ErrorPort=off  RemotePort=off  LengthPort=off  StatusPort=off  ApplyMinMax=off
      settings: SourceProductBaseCode=ME,XP,VN  DataFormat=raw data
  Constant4 : Constant  OutDataTypeStr=boolean
  Data Store Read1 : DataStoreRead  DataStoreName=CAN_trm  DataStoreElements=CAN_trm.wCCacc  IndexOptions=Index vector (dialog)  Indices=1  OutputSizes=1
  Data Store Read2 : DataStoreRead  DataStoreName=CAN_trm  DataStoreElements=CAN_trm.wCCcoast  IndexOptions=Index vector (dialog)  Indices=1  OutputSizes=1
  Data Store Read3 : DataStoreRead  DataStoreName=CAN_trm  DataStoreElements=CAN_trm.wCCresume  IndexOptions=Index vector (dialog)  Indices=1  OutputSizes=1
  Data Store Read4 : DataStoreRead  DataStoreName=CAN_trm  DataStoreElements=CAN_trm.wCCset  IndexOptions=Index vector (dialog)  Indices=1  OutputSizes=1
  Data Store Read5 : DataStoreRead  DataStoreName=in_stats  DataStoreElements=in_stats.inCCacc  IndexOptions=Index vector (dialog)  Indices=1  OutputSizes=1
  Data Store Read6 : DataStoreRead  DataStoreName=in_stats  DataStoreElements=in_stats.inCCcoast  IndexOptions=Index vector (dialog)  Indices=1  OutputSizes=1
  Data Store Read7 : DataStoreRead  DataStoreName=in_stats  DataStoreElements=in_stats.inCCresume  IndexOptions=Index vector (dialog)  Indices=1  OutputSizes=1
  Data Store Read8 : DataStoreRead  DataStoreName=in_stats  DataStoreElements=in_stats.inCCset  IndexOptions=Index vector (dialog)  Indices=1  OutputSizes=1
  Data Store Write : DataStoreWrite  DataStoreName=CAN_transm_stat  DataStoreElements=CAN_transm_stat(10)  IndexOptions=Index vector (dialog)  Indices=1  OutputSizes=1
  FCAN_Send : mbd_mpc574x_ec_toolbox/Communication Blocks/CAN Blocks/FCAN_Send  Priority=2  can_instance=0  can_mode=Non-blocking  can_timeout_ms=0  can_mb_idx=10  can_extended_id=on  can_is_remote=off  can_id=0CFEF111  show_adv_opts=on  can_fd_enable=off  can_enable_brs=off  can_fd_padding=0
      settings: SourceProductName=NXP Model-Based Design Toolbox for MPC57xx MCUs
  OR{,1..3} (4 alike) : Logic  Operator=OR  AllPortsSameDT=off  OutDataTypeStr=boolean
  Width : Width  DataType=uint8
  wires:
  Data Store Read4/1 -> OR3/1
  Data Store Read8/1 -> OR3/2
  Data Store Read7/1 -> OR2/2
  Data Store Read3/1 -> OR2/1
  Data Store Read2/1 -> OR1/1
  Data Store Read6/1 -> OR1/2
  Data Store Read5/1 -> OR/2
  Data Store Read1/1 -> OR/1
  OR3/1 -> CAN Pack/4
  OR2/1 -> CAN Pack/3
  OR1/1 -> CAN Pack/2
  OR/1 -> CAN Pack/1
  Width/1 -> FCAN_Send/2
  Constant4/1 -> Data Store Write/1
  CAN Unpack/1 -> Width/1, FCAN_Send/1
  CAN Pack/1 -> CAN Unpack/1

== system BCM2_4/CAN0 Transmit buf 5-21/0x18FEF461 Чтение//Запись EEPROM buf = 6/EBC1 0x18F0010B buf = 6 ==
  CAN Pack : canmsglib/CAN Pack  MsgList=(none)  MsgName=EEPROM_RW  MsgIDType=Extended (29-bit identifier)  MsgIdentifier=hex2dec('18FEF461')  MsgLength=8  Remote=off  ApplyMinMax=off  BusOutput=off  SignalInfo={ 'CMD', '0', '8', 'LE', 'unsigned', 'Standard', '0', '1', '0', '-Inf', 'Inf'; 'Adress', '8', '8', 'LE', 'unsigned', 'Standard', '0', '1', '0', '-Inf', 'Inf'; 'Data', '16', '16', 'LE', 'unsigned', 'Standard', '0', '1', '0', '-Inf', 'Inf' }
      settings: SourceProductBaseCode=ME,XP,VN  DataFormat=manually specified signals
  CAN Unpack : canmsglib/CAN Unpack  MsgList=(none)  MsgName=CAN Msg  MsgIDType=Extended (29-bit identifier)  MsgIdentifier=hex2dec('18FEF461')  MsgLength=8  SignalInfo={}  IDPort=off  TimestampPort=off  ErrorPort=off  RemotePort=off  LengthPort=off  StatusPort=off  ApplyMinMax=off
      settings: SourceProductBaseCode=ME,XP,VN  DataFormat=raw data
  Constant1 : Constant  Value=0  OutDataTypeStr=boolean
  Constant4 : Constant  OutDataTypeStr=boolean
  Data Store Read : DataStoreRead  DataStoreName=CAN_trm  DataStoreElements=CAN_trm.ee_cmd#CAN_trm.ee_adr#CAN_trm.ee_data  IndexOptions=Index vector (dialog)  Indices=1  OutputSizes=1
  Data Store Write : DataStoreWrite  DataStoreName=CAN_transm_stat  DataStoreElements=CAN_transm_stat(6)  IndexOptions=Index vector (dialog)  Indices=1  OutputSizes=1
  Data Store Write1 : DataStoreWrite  DataStoreName=CAN_trm  DataStoreElements=CAN_trm.ee_en_trm  IndexOptions=Index vector (dialog)  Indices=1  OutputSizes=1
  FCAN_Send : mbd_mpc574x_ec_toolbox/Communication Blocks/CAN Blocks/FCAN_Send  Priority=2  can_instance=0  can_mode=Non-blocking  can_timeout_ms=0  can_mb_idx=6  can_extended_id=on  can_is_remote=off  can_id=18FEF461  show_adv_opts=on  can_fd_enable=off  can_enable_brs=off  can_fd_padding=0
      settings: SourceProductName=NXP Model-Based Design Toolbox for MPC57xx MCUs
  Width : Width  DataType=uint8
  wires:
  Constant4/1 -> Data Store Write/1
  Width/1 -> FCAN_Send/2
  Constant1/1 -> Data Store Write1/1
  CAN Pack/1 -> CAN Unpack/1
  CAN Unpack/1 -> Width/1, FCAN_Send/1
  Data Store Read/1 -> CAN Pack/1
  Data Store Read/2 -> CAN Pack/2
  Data Store Read/3 -> CAN Pack/3

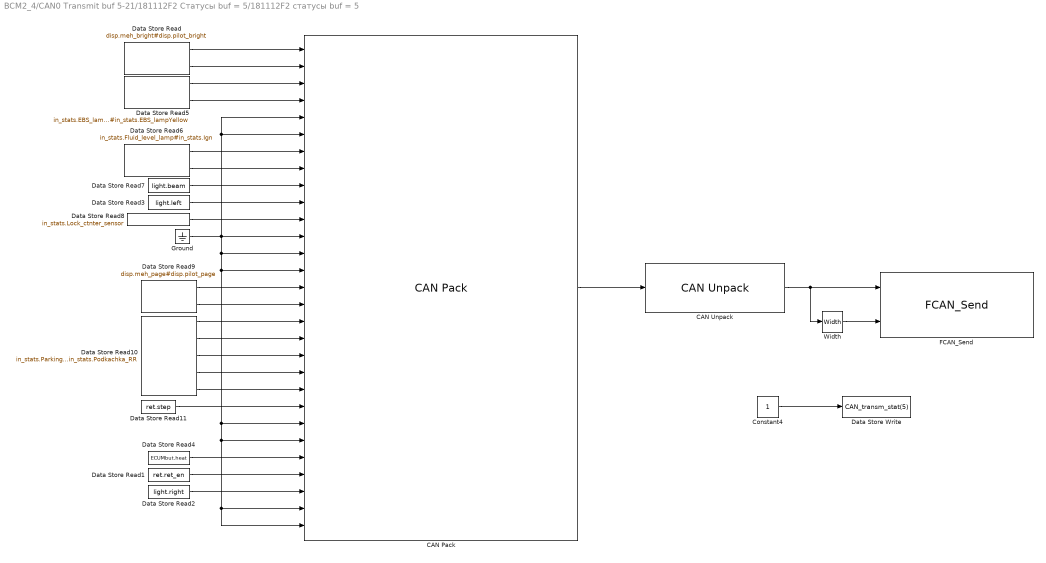
== system BCM2_4/CAN0 Transmit buf 5-21/181112F2 Статусы buf = 5/181112F2 статусы buf = 5 ==
  CAN Pack : canmsglib/CAN Pack  CANdbFile=C:\Users\km-dea\Desktop\KAMAZ_master_full.dbc  MsgList=K73_status  MsgName=K73_status  MsgIDType=Extended (29-bit identifier)  MsgIdentifier=403772146  MsgLength=8  Remote=off  ApplyMinMax=off  BusOutput=off  SignalInfo={'Bright_mehanic','24','8','LE','unsigned','Standard','0','1','0','-Inf','Inf';'Bright_pilot','16','8','LE','unsigned','Standard','0','1','0','-Inf','Inf';'EBS_lamp_red','55','1','LE','unsigned','Standard','0','1','0','-Inf','Inf';'EBS_lamp_yellow','54','1','LE','unsigned','Standard','0','1','0','-Inf','Inf';'Err_fuel_pump1','47','1','LE','unsigned','Standard','0','1','0','-Inf','Inf';'Err_fuel_pump2','48','1','LE','unsigned','Standard','0','1','0','-Inf','Inf';'Fluid_level_lamp','61','1','LE','unsigned','Standard','0','1','0','-Inf','Inf';'IGN_stat','41','1','LE','unsigned','Standard','0','1','0','-Inf','Inf';'Lamp_beam','60','1','LE','unsigned','Standard','0','1','0','-Inf','Inf';'Left_turn','58','1','LE','unsigned','Standard','0','1','0','-Inf','Inf';'Lock_center_sensor','57','1','LE','unsigned','Standard','0','1','0','-Inf','Inf';'Lock_crnter_out','49','1','LE','unsigned','Standard','0','1','0','-Inf','Inf';'Lock_front_out','56','1','LE','unsigned','Standard','0','1','0','-Inf','Inf';'Lock_rear_sensor','63','1','LE','unsigned','Standard','0','1','0','-Inf','Inf';'Page_mehanic','8','8','LE','unsigned','Standard','0','1','0','-Inf','Inf';'Page_pilot','0','8','LE','unsigned','Standard','0','1','0','-Inf','Inf';'Parking_lamp','62','1','LE','unsigned','Standard','0','1','0','-Inf','Inf';'Podkachka_FL','50','1','LE','unsigned','Standard','0','1','0','-Inf','Inf';'Podkachka_FR','51','1','LE','unsigned','Standard','0','1','0','-Inf','Inf';'Podkachka_RL','52','1','LE','unsigned','Standard','0','1','0','-Inf','Inf';'Podkachka_RR','53','1','LE','unsigned','Standard','0','1','0','-Inf','Inf';'Reatarder_step','32','8','LE','unsigned','Standard','0','1','0','-Inf','Inf';'Rele_fuel_pump1','45','1','LE','unsigned','Standard','0','1','0','-Inf','Inf';'Rele_fuel_pump2','46','1','LE','unsigned','Standard','0','1','0','-Inf','Inf';'Rele_heat_glass','44','1','LE','unsigned','Standard','0','1','0','-Inf','Inf';'Retarder_stat','40','1','LE','unsigned','Standard','0','1','0','-Inf','Inf';'Right_turn','59','1','LE','unsigned','Standard','0','1','0','-Inf','Inf';'Stab_front','43','1','LE','unsigned','Standard','0','1','0','-Inf','Inf';'Stab_rear','42','1','LE','unsigned','Standard','0','1','0','-Inf','Inf'}
      settings: SourceProductBaseCode=ME,XP,VN  DataFormat=CANdb specified signals
  CAN Unpack : canmsglib/CAN Unpack  MsgList=(none)  MsgName=CAN Msg  MsgIDType=Extended (29-bit identifier)  MsgIdentifier=403772146  MsgLength=8  SignalInfo={}  IDPort=off  TimestampPort=off  ErrorPort=off  RemotePort=off  LengthPort=off  StatusPort=off  ApplyMinMax=off
      settings: SourceProductBaseCode=ME,XP,VN  DataFormat=raw data
  Constant4 : Constant  OutDataTypeStr=boolean
  Data Store Read : DataStoreRead  DataStoreName=disp  DataStoreElements=disp.meh_bright#disp.pilot_bright  IndexOptions=Index vector (dialog)  Indices=1  OutputSizes=1
  Data Store Read1 : DataStoreRead  DataStoreName=ret  DataStoreElements=ret.ret_en  IndexOptions=Index vector (dialog)  Indices=1  OutputSizes=1
  Data Store Read10 : DataStoreRead  DataStoreName=in_stats  DataStoreElements=in_stats.Parking_brake#in_stats.Podkachka_FL#in_stats.Podkachka_FR#in_stats.Podkachka_RL#in_stats.Podkachka_RR  IndexOptions=Index vector (dialog)  Indices=1  OutputSizes=1
  Data Store Read11 : DataStoreRead  DataStoreName=ret  DataStoreElements=ret.step  IndexOptions=Index vector (dialog)  Indices=1  OutputSizes=1
  Data Store Read2 : DataStoreRead  DataStoreName=light  DataStoreElements=light.right  IndexOptions=Index vector (dialog)  Indices=1  OutputSizes=1
  Data Store Read3 : DataStoreRead  DataStoreName=light  DataStoreElements=light.left  IndexOptions=Index vector (dialog)  Indices=1  OutputSizes=1
  Data Store Read4 : DataStoreRead  DataStoreName=ECUMbut  DataStoreElements=ECUMbut.heat  IndexOptions=Index vector (dialog)  Indices=1  OutputSizes=1
  Data Store Read5 : DataStoreRead  DataStoreName=in_stats  DataStoreElements=in_stats.EBS_lampRED#in_stats.EBS_lampYellow  IndexOptions=Index vector (dialog)  Indices=1  OutputSizes=1
  Data Store Read6 : DataStoreRead  DataStoreName=in_stats  DataStoreElements=in_stats.Fluid_level_lamp#in_stats.Ign  IndexOptions=Index vector (dialog)  Indices=1  OutputSizes=1
  Data Store Read7 : DataStoreRead  DataStoreName=light  DataStoreElements=light.beam  IndexOptions=Index vector (dialog)  Indices=1  OutputSizes=1
  Data Store Read8 : DataStoreRead  DataStoreName=in_stats  DataStoreElements=in_stats.Lock_ctnter_sensor  IndexOptions=Index vector (dialog)  Indices=1  OutputSizes=1
  Data Store Read9 : DataStoreRead  DataStoreName=disp  DataStoreElements=disp.meh_page#disp.pilot_page  IndexOptions=Index vector (dialog)  Indices=1  OutputSizes=1
  Data Store Write : DataStoreWrite  DataStoreName=CAN_transm_stat  DataStoreElements=CAN_transm_stat(5)  IndexOptions=Index vector (dialog)  Indices=1  OutputSizes=1
  FCAN_Send : mbd_mpc574x_ec_toolbox/Communication Blocks/CAN Blocks/FCAN_Send  Priority=2  can_instance=0  can_mode=Non-blocking  can_timeout_ms=0  can_mb_idx=5  can_extended_id=on  can_is_remote=off  can_id=181112F2  show_adv_opts=on  can_fd_enable=off  can_enable_brs=off  can_fd_padding=0
      settings: SourceProductName=NXP Model-Based Design Toolbox for MPC57xx MCUs
  Ground : Ground
  Width : Width  DataType=uint8
  wires:
  Width/1 -> FCAN_Send/2
  Constant4/1 -> Data Store Write/1
  CAN Unpack/1 -> Width/1, FCAN_Send/1
  CAN Pack/1 -> CAN Unpack/1
  Data Store Read/1 -> CAN Pack/1
  Data Store Read/2 -> CAN Pack/2
  Ground/1 -> CAN Pack/23, CAN Pack/24, CAN Pack/28, CAN Pack/29, CAN Pack/14, CAN Pack/13, CAN Pack/5, CAN Pack/6, CAN Pack/12
  Data Store Read1/1 -> CAN Pack/26
  Data Store Read2/1 -> CAN Pack/27
  Data Store Read3/1 -> CAN Pack/10
  Data Store Read4/1 -> CAN Pack/25
  Data Store Read5/2 -> CAN Pack/4
  Data Store Read5/1 -> CAN Pack/3
  Data Store Read6/1 -> CAN Pack/7
  Data Store Read6/2 -> CAN Pack/8
  Data Store Read7/1 -> CAN Pack/9
  Data Store Read8/1 -> CAN Pack/11
  Data Store Read9/1 -> CAN Pack/15
  Data Store Read9/2 -> CAN Pack/16
  Data Store Read10/1 -> CAN Pack/17
  Data Store Read10/2 -> CAN Pack/18
  Data Store Read10/3 -> CAN Pack/19
  Data Store Read10/4 -> CAN Pack/20
  Data Store Read10/5 -> CAN Pack/21
  Data Store Read11/1 -> CAN Pack/22

== system BCM2_4/CAN0 Transmit buf 5-21/18F0010B buf = 7/18F0010B buf = 7 ==
  Constant4 : Constant  OutDataTypeStr=boolean
  Data Store Read : DataStoreRead  DataStoreName=CAN_rec  DataStoreElements=CAN_rec.m18F0010B(:)  IndexOptions=Index vector (dialog)  Indices=1  OutputSizes=1
  Data Store Write : DataStoreWrite  DataStoreName=CAN_transm_stat  DataStoreElements=CAN_transm_stat(7)  IndexOptions=Index vector (dialog)  Indices=1  OutputSizes=1
  FCAN_Send : mbd_mpc574x_ec_toolbox/Communication Blocks/CAN Blocks/FCAN_Send  Priority=2  can_instance=0  can_mode=Non-blocking  can_timeout_ms=0  can_mb_idx=7  can_extended_id=on  can_is_remote=off  can_id=18F0010B  show_adv_opts=on  can_fd_enable=off  can_enable_brs=off  can_fd_padding=0
      settings: SourceProductName=NXP Model-Based Design Toolbox for MPC57xx MCUs
  Width : Width  DataType=uint8
  wires:
  Data Store Read/1 -> FCAN_Send/1, Width/1
  Constant4/1 -> Data Store Write/1
  Width/1 -> FCAN_Send/2

== system BCM2_4/CAN0 Transmit buf 5-21/18FEAD0B buf = 8/18FEAD0B buf = 8 ==
  Constant4 : Constant  OutDataTypeStr=boolean
  Data Store Read : DataStoreRead  DataStoreName=CAN_rec  DataStoreElements=CAN_rec.m18FEAD0B(:)  IndexOptions=Index vector (dialog)  Indices=1  OutputSizes=1
  Data Store Write : DataStoreWrite  DataStoreName=CAN_transm_stat  DataStoreElements=CAN_transm_stat(8)  IndexOptions=Index vector (dialog)  Indices=1  OutputSizes=1
  FCAN_Send : mbd_mpc574x_ec_toolbox/Communication Blocks/CAN Blocks/FCAN_Send  Priority=2  can_instance=0  can_mode=Non-blocking  can_timeout_ms=0  can_mb_idx=8  can_extended_id=on  can_is_remote=off  can_id=18FEAD0B  show_adv_opts=on  can_fd_enable=off  can_enable_brs=off  can_fd_padding=0
      settings: SourceProductName=NXP Model-Based Design Toolbox for MPC57xx MCUs
  Width : Width  DataType=uint8
  wires:
  Width/1 -> FCAN_Send/2
  Constant4/1 -> Data Store Write/1
  Data Store Read/1 -> Width/1, FCAN_Send/1
